simulink model "backups"  (R2024a)
settings: Solver=VariableStepAuto  StartTime=0.0  StopTime=10.0  RelTol=1e-3
values from neighbouring files (symbols this model uses):
  AttKd_x = inp(4,2).Var2    [SFF_Simulator_Entradas.m]
  AttKd_y = inp(5,2).Var2    [SFF_Simulator_Entradas.m]
  AttKd_z = inp(6,2).Var2    [SFF_Simulator_Entradas.m]
  AttKp_x = inp(1,2).Var2    [SFF_Simulator_Entradas.m]
  AttKp_y = inp(2,2).Var2    [SFF_Simulator_Entradas.m]
  AttKp_z = inp(3,2).Var2    [SFF_Simulator_Entradas.m]
  B = inp(8,2).Var2    [SFF_Simulator_Entradas.m]
  beta = inp(2,2).Var2    [SFF_Simulator_Entradas.m]
  Cd1 = inp(4,2).Var2    [SFF_Simulator_Entradas.m]
  cdgps = inp(1,2).Var2    [SFF_Simulator_Entradas.m]
  estrelas = inp(4,2).Var2    [SFF_Simulator_Entradas.m]
  estrelas_bias = inp(6,2).Var2    [SFF_Simulator_Entradas.m]
  estrelas_ruido = inp(5,2).Var2    [SFF_Simulator_Entradas.m]
  Fn = inp(2,2).Var2    [SFF_Simulator_Entradas.m]
  gps_bias = inp(3,2).Var2    [SFF_Simulator_Entradas.m]
  gps_ruido = inp(2,2).Var2    [SFF_Simulator_Entradas.m]
  Iw = inp(7,2).Var2    [SFF_Simulator_Entradas.m]
  Ixx = inp(7,2).Var2    [SFF_Simulator_Entradas.m]
  Iyy = inp(8,2).Var2    [SFF_Simulator_Entradas.m]
  Izz = inp(9,2).Var2    [SFF_Simulator_Entradas.m]
  Km = inp(3,2).Var2    [SFF_Simulator_Entradas.m]
  Kv = inp(9,2).Var2    [SFF_Simulator_Entradas.m]
  L1 = inp(5,2).Var2    [SFF_Simulator_Entradas.m]
  limCorrente = inp(4,2).Var2    [SFF_Simulator_Entradas.m]
  limVolt = inp(5,2).Var2    [SFF_Simulator_Entradas.m]
  m1 = inp(6,2).Var2    [SFF_Simulator_Entradas.m]
  magne = inp(10,2).Var2    [SFF_Simulator_Entradas.m]
  magne_bias = inp(12,2).Var2    [SFF_Simulator_Entradas.m]
  magne_ruido = inp(11,2).Var2    [SFF_Simulator_Entradas.m]
  man = inp(1,2).Var2    [SFF_Simulator_Entradas.m]
  OrbKd_x = inp(3,2).Var2    [SFF_Simulator_Entradas.m]
  OrbKd_y = inp(6,2).Var2    [SFF_Simulator_Entradas.m]
  OrbKd_z = inp(9,2).Var2    [SFF_Simulator_Entradas.m]
  OrbKi_x = inp(2,2).Var2    [SFF_Simulator_Entradas.m]
  OrbKi_y = inp(5,2).Var2    [SFF_Simulator_Entradas.m]
  OrbKi_z = inp(8,2).Var2    [SFF_Simulator_Entradas.m]
  OrbKp_x = inp(1,2).Var2    [SFF_Simulator_Entradas.m]
  OrbKp_y = inp(4,2).Var2    [SFF_Simulator_Entradas.m]
  OrbKp_z = inp(7,2).Var2    [SFF_Simulator_Entradas.m]
  propForcaAtivo = inp(1,2).Var2    [SFF_Simulator_Entradas.m]
  Rm = inp(6,2).Var2    [SFF_Simulator_Entradas.m]
  rodaAtivo = inp(1,2).Var2    [SFF_Simulator_Entradas.m]
  RodKi = inp(1,2).Var2    [SFF_Simulator_Entradas.m]
  sat_torquerod = inp(14,2).Var2    [SFF_Simulator_Entradas.m]
  torqrodAtivo = inp(1,2).Var2    [SFF_Simulator_Entradas.m]
undefined symbols (not defined in the file or in its folder): IAU, J2, mi, omega_E, propMomentoAtivo, Re, sat_rodareacao, WMM2020
libraries: dspsrcs4 x19, aerolibtransform2 x2, aerolibgravity2 x2, simulink x1
(part 3 of 4)

== system backups/Atuadores de Atitude/Atuador atitude ativado ==
  note: Entradas
  note: Atuador atitude ativado
  note: Saídas
  MtsProp : Inport
  Mts : Inport  Port=2
  dinCinOrb : Inport  Port=3
  A_q : Inport  Port=4
  Action Port : ActionPort  ActionPortLabel=if(u1 > 0)
  Bus Selector : BusSelector  OutputSignals=T_In_LVLH,r1_vec_I
  Cast To Single : DataTypeConversion  OutDataTypeStr=single  SaturateOnIntegerOverflow=off  RndMeth=Floor
  Cast To Single1 : DataTypeConversion  OutDataTypeStr=single  SaturateOnIntegerOverflow=off  RndMeth=Floor
  Cast To Single2 : DataTypeConversion  OutDataTypeStr=single  SaturateOnIntegerOverflow=off  RndMeth=Floor
  Constant4 : Constant  Value=rodaAtivo  SampleTime=-1
  Constant5 : Constant  Value=propForcaAtivo  SampleTime=-1
  Constant9 : Constant  Value=torqrodAtivo  SampleTime=-1
  If : If  NumInputs=3  IfExpression=u1 > 0 & u2 == 0 & u3 == 0  ElseIfExpressions=u2 > 0, u3 > 0  ShowElse=off
  Magnetorquer ativado : Subsystem  TreatAsAtomicUnit=on
  Merge : Merge  Inputs=3
  Propulsor ativado : Subsystem  TreatAsAtomicUnit=on
  Rodas de reação ativadas : Subsystem  TreatAsAtomicUnit=on
  MtsReal : Outport
  wires:
  Bus Selector/2 -> [r1_vec_I]  "<r1_vec_I>"
  Bus Selector/1 -> [T_In_LVLH]  "<T_In_LVLH>"
  dinCinOrb/1 -> Bus Selector/1
  If/1 -> Propulsor ativado/Action
  Propulsor ativado/1(Out1) -> Merge/1
  Rodas de reação ativadas/1(TcReal_rodareacao) -> Merge/2
  Magnetorquer ativado/1(TcReal_torqrod_roda) -> Merge/3
  If/3 -> Magnetorquer ativado/Action
  MtsProp/1 -> [MtsProp]
  Mts/1 -> [Mts]
  A_q/1 -> [A_q]
  Merge/1 -> [MtsReal]
  [MtsReal] -> MtsReal/1
  Constant9/1 -> Cast To Single2/1
  Cast To Single1/1 -> If/2
  Cast To Single2/1 -> If/3
  Constant4/1 -> Cast To Single1/1
  Cast To Single/1 -> If/1
  Constant5/1 -> Cast To Single/1
  [MtsProp] -> Propulsor ativado/1(In1)
  [Mts] -> Rodas de reação ativadas/1(Tc)
  If/2 -> Rodas de reação ativadas/Action
  [MtsProp] -> Rodas de reação ativadas/2(MtsProp)
  [A_q] -> Magnetorquer ativado/3(A_q)
  [T_In_LVLH] -> Magnetorquer ativado/2(T_In_LVLH)
  [r1_vec_I] -> Magnetorquer ativado/4(r1_vec_I)
  [Mts] -> Magnetorquer ativado/1(Tc)
  [MtsProp] -> Magnetorquer ativado/5(MtsProp)

== system backups/Atuadores de Atitude/Atuador atitude desativado ==
  In1 : Inport
  Action Port : ActionPort  ActionPortLabel=else
  Out1 : Outport
  wires:
  In1/1 -> Out1/1

== system backups/Atuadores de Atitude1/Atuador atitude ativado ==
  note: Entradas
  note: Atuador atitude ativado
  note: Saídas
  MtsProp : Inport
  Mts : Inport  Port=2
  dinCinOrb : Inport  Port=3
  A_q : Inport  Port=4
  Action Port : ActionPort
  Bus Selector : BusSelector  OutputSignals=T_In_LVLH,r1_vec_I
  Cast To Single : DataTypeConversion  OutDataTypeStr=single  SaturateOnIntegerOverflow=off  RndMeth=Floor
  Cast To Single1 : DataTypeConversion  OutDataTypeStr=single  SaturateOnIntegerOverflow=off  RndMeth=Floor
  Cast To Single2 : DataTypeConversion  OutDataTypeStr=single  SaturateOnIntegerOverflow=off  RndMeth=Floor
  Constant4 : Constant  Value=rodaAtivo  SampleTime=-1
  Constant5 : Constant  Value=propForcaAtivo  SampleTime=-1
  Constant9 : Constant  Value=torqrodAtivo  SampleTime=-1
  If : If  NumInputs=3  IfExpression=u1 > 0 & u2 == 0 & u3 == 0  ElseIfExpressions=u2 > 0, u3 > 0  ShowElse=off
  Magnetorquer ativado : Subsystem  TreatAsAtomicUnit=on
  Merge : Merge  Inputs=3
  Propulsor ativado : Subsystem  TreatAsAtomicUnit=on
  Rodas de reação ativadas : Subsystem  TreatAsAtomicUnit=on
  MtsReal : Outport
  wires:
  Bus Selector/2 -> [r1_vec_I]  "<r1_vec_I>"
  Bus Selector/1 -> [T_In_LVLH]  "<T_In_LVLH>"
  dinCinOrb/1 -> Bus Selector/1
  Constant5/1 -> Cast To Single/1
  Cast To Single/1 -> If/1
  Constant4/1 -> Cast To Single1/1
  Constant9/1 -> Cast To Single2/1
  Cast To Single1/1 -> If/2
  Cast To Single2/1 -> If/3
  If/1 -> Propulsor ativado/Action
  If/2 -> Rodas de reação ativadas/Action
  Propulsor ativado/1(Out1) -> Merge/1
  Rodas de reação ativadas/1(TcReal_rodareacao) -> Merge/2
  Magnetorquer ativado/1(TcReal_torqrod_roda) -> Merge/3
  If/3 -> Magnetorquer ativado/Action
  MtsProp/1 -> [MtsProp]
  [MtsProp] -> Propulsor ativado/1(In1)
  Mts/1 -> [Mts]
  [Mts] -> Magnetorquer ativado/1(Tc)
  [T_In_LVLH] -> Magnetorquer ativado/2(T_In_LVLH)
  [r1_vec_I] -> Magnetorquer ativado/4(r1_vec_I)
  [A_q] -> Magnetorquer ativado/3(A_q)
  A_q/1 -> [A_q]
  Merge/1 -> [MtsReal]
  [MtsReal] -> MtsReal/1
  [Mts] -> Rodas de reação ativadas/1(Tc)
  [MtsProp] -> Rodas de reação ativadas/2(MtsProp)
  [MtsProp] -> Magnetorquer ativado/5(MtsProp)

== system backups/Atuadores de Atitude1/Atuador atitude desativado ==
  In1 : Inport
  Action Port : ActionPort
  Out1 : Outport
  wires:
  In1/1 -> Out1/1

== system backups/Sensores Atitude/Sensor ativado ==
  atitudeIn : Inport
  Action Port : ActionPort
  Demux : Demux  Outputs=3
  Mux : Mux  Inputs=3
  estrelasSensor_phi : Subsystem
  estrelasSensor_psi : Subsystem
  estrelasSensor_theta : Subsystem
  atitudeOut : Outport
  wires:
  Demux/3 -> estrelasSensor_psi/1(In1)
  Demux/2 -> estrelasSensor_theta/1(In1)
  Demux/1 -> estrelasSensor_phi/1(phiIn)
  atitudeIn/1 -> Demux/1
  estrelasSensor_phi/1(phiOut) -> Mux/1
  estrelasSensor_theta/1(Out1) -> Mux/2
  estrelasSensor_psi/1(Out1) -> Mux/3
  Mux/1 -> atitudeOut/1

== system backups/Sensores Atitude/Sensor desativado ==
  atitudeIn : Inport
  Action Port : ActionPort
  atitudeOut : Outport
  wires:
  atitudeIn/1 -> atitudeOut/1

== system backups/Sensores Atitude1/Sensor ativado ==
  atitude : Inport
  Action Port : ActionPort
  Demux : Demux  Outputs=3
  Mux : Mux  Inputs=3
  estrelasSensor_phi : Subsystem
  estrelasSensor_psi : Subsystem
  estrelasSensor_theta : Subsystem
  atitudeSen : Outport
  wires:
  Demux/3 -> estrelasSensor_psi/1(In1)
  Demux/2 -> estrelasSensor_theta/1(In1)
  Demux/1 -> estrelasSensor_phi/1(In1)
  atitude/1 -> Demux/1
  estrelasSensor_phi/1(Out1) -> Mux/1  "x"
  estrelasSensor_theta/1(Out1) -> Mux/2  "y"
  estrelasSensor_psi/1(Out1) -> Mux/3  "z"
  Mux/1 -> atitudeSen/1

== system backups/Sensores Atitude1/Sensor desativado ==
  atitude : Inport
  Action Port : ActionPort
  atitudeSen : Outport
  wires:
  atitude/1 -> atitudeSen/1

== system backups/Sensores Orbital/Sensor ativado ==
  dinCinOrbIn : Inport
  Action Port : ActionPort
  Bus Creator : BusCreator  Inputs=18
  Bus Selector : BusSelector  OutputSignals=x,y,z
  Bus Selector1 : BusSelector  OutputSignals=x_dot,y_dot,z_dot,r0,omega_x,omega_y,omega_z,omega_x_dot,omega_y_dot,omega_z_dot,T_In_LVLH,r1_vec_I,i1,ohm1,theta1
  GPSsensor : Subsystem
  GPSsensor1 : Subsystem
  GPSsensor2 : Subsystem
  dinCinOrbOut : Outport
  wires:
  Bus Selector/3 -> GPSsensor2/1(In1)  "<z>"
  Bus Selector/2 -> GPSsensor1/1(In1)  "<y>"
  Bus Selector/1 -> GPSsensor/1(In1)  "<x>"
  dinCinOrbIn/1 -> Bus Selector/1, Bus Selector1/1
  Bus Creator/1 -> dinCinOrbOut/1
  Bus Selector1/4 -> Bus Creator/7  "<r0>"
  Bus Selector1/5 -> Bus Creator/8  "<omega_x>"
  Bus Selector1/6 -> Bus Creator/9  "<omega_y>"
  Bus Selector1/7 -> Bus Creator/10  "<omega_z>"
  Bus Selector1/8 -> Bus Creator/11  "<omega_x_dot>"
  Bus Selector1/9 -> Bus Creator/12  "<omega_y_dot>"
  Bus Selector1/10 -> Bus Creator/13  "<omega_z_dot>"
  Bus Selector1/11 -> Bus Creator/14  "<T_In_LVLH>"
  Bus Selector1/12 -> Bus Creator/15  "<r1_vec_I>"
  Bus Selector1/13 -> Bus Creator/16  "<i1>"
  Bus Selector1/14 -> Bus Creator/17  "<ohm1>"
  Bus Selector1/15 -> Bus Creator/18  "<theta1>"
  GPSsensor2/1(Out1) -> Bus Creator/5  "z"
  GPSsensor1/1(Out1) -> Bus Creator/3  "y"
  GPSsensor/1(Out1) -> Bus Creator/1  "x"
  Bus Selector1/1 -> Bus Creator/2  "<x_dot>"
  Bus Selector1/2 -> Bus Creator/4  "<y_dot>"
  Bus Selector1/3 -> Bus Creator/6  "<z_dot>"

== system backups/Sensores Orbital/Sensor desativado ==
  dinCinOrbIn : Inport
  Action Port : ActionPort
  dinCinOrbOut : Outport
  wires:
  dinCinOrbIn/1 -> dinCinOrbOut/1

== system backups/Sensores Orbital1/Sensor ativado ==
  dinCinOrb : Inport
  Action Port : ActionPort
  Bus Creator : BusCreator  Inputs=18
  Bus Selector : BusSelector  OutputSignals=x,y,z
  Bus Selector1 : BusSelector  OutputSignals=x_dot,y_dot,z_dot,r0,omega_x,omega_y,omega_z,omega_x_dot,omega_y_dot,omega_z_dot,T_In_LVLH,r1_vec_I,i1,ohm1,theta1
  GPSsensor : Subsystem
  GPSsensor1 : Subsystem
  GPSsensor2 : Subsystem
  Out1 : Outport
  wires:
  Bus Selector/3 -> GPSsensor2/1(In1)  "<z>"
  Bus Selector/2 -> GPSsensor1/1(In1)  "<y>"
  Bus Selector/1 -> GPSsensor/1(In1)  "<x>"
  dinCinOrb/1 -> Bus Selector/1, Bus Selector1/1
  Bus Creator/1 -> Out1/1
  Bus Selector1/4 -> Bus Creator/7  "<r0>"
  Bus Selector1/5 -> Bus Creator/8  "<omega_x>"
  Bus Selector1/6 -> Bus Creator/9  "<omega_y>"
  Bus Selector1/7 -> Bus Creator/10  "<omega_z>"
  Bus Selector1/8 -> Bus Creator/11  "<omega_x_dot>"
  Bus Selector1/9 -> Bus Creator/12  "<omega_y_dot>"
  Bus Selector1/10 -> Bus Creator/13  "<omega_z_dot>"
  Bus Selector1/11 -> Bus Creator/14  "<T_In_LVLH>"
  Bus Selector1/12 -> Bus Creator/15  "<r1_vec_I>"
  Bus Selector1/13 -> Bus Creator/16  "<i1>"
  Bus Selector1/14 -> Bus Creator/17  "<ohm1>"
  Bus Selector1/15 -> Bus Creator/18  "<theta1>"
  GPSsensor2/1(Out1) -> Bus Creator/5  "z"
  GPSsensor1/1(Out1) -> Bus Creator/3  "y"
  GPSsensor/1(Out1) -> Bus Creator/1  "x"
  Bus Selector1/1 -> Bus Creator/2  "<x_dot>"
  Bus Selector1/2 -> Bus Creator/4  "<y_dot>"
  Bus Selector1/3 -> Bus Creator/6  "<z_dot>"

== system backups/Sensores Orbital1/Sensor desativado ==
  dinCinOrb : Inport
  Action Port : ActionPort
  Out1 : Outport
  wires:
  dinCinOrb/1 -> Out1/1

== system backups/atuadoresAtitude/conjunto2TorqRods1RodaReacao ==
  Tc : Inport
  T_In_LVLH : Inport  Port=2
  A_q : Inport  Port=3
  r1_vec_I : Inport  Port=4
  Constant9 : Constant  Value=torqrodAtivo  SampleTime=-1
  Demux1 : Demux  Outputs=3
  ECI Position to LLA : aerolibtransform2/ECI Position to LLA  red=IAU-2000/2006  year=2013  month=January  day=1  hour=0  min=0  sec=0  deltaT=None  errorflag=Error  extraparamflag=off  eunits=Metric (MKS)  earthmodel=WGS84  flat=1/298.257223563  eqradius=6378137
      settings: AttributesFormatString=%<red>
  Gain : Gain  Gain=pi/180
  Gain1 : Gain  Gain=pi/180
  HardwareDeControle (Rodas de Reação + 2 Torqrods) : Subsystem
  If : If
  If Action Subsystem : Subsystem  TreatAsAtomicUnit=on
  If Action Subsystem1 : Subsystem  TreatAsAtomicUnit=on
  Merge : Merge
  Product : Product  Multiplication=Matrix(*)
  Product1 : Product  Multiplication=Matrix(*)
  TcReal_torqrod_roda : Outport
  wires:
  HardwareDeControle (Rodas de Reação + 2 Torqrods)/1(Tc fornecido) -> TcReal_torqrod_roda/1
  Tc/1 -> HardwareDeControle (Rodas de Reação + 2 Torqrods)/1(Tc)
  T_In_LVLH/1 -> Product/1
  Product/1 -> Product1/2
  Product1/1 -> HardwareDeControle (Rodas de Reação + 2 Torqrods)/2(B_seg)  "B_seg"
  A_q/1 -> Product1/1
  Constant9/1 -> [torqrodAtivo]
  [torqrodAtivo] -> If/1
  If/1 -> If Action Subsystem/Action
  [lonSeg] -> If Action Subsystem/3(lonSeg)
  [altSeg] -> If Action Subsystem/1(altSeg)
  [latSeg] -> If Action Subsystem/2(latSeg)
  If/2 -> If Action Subsystem1/Action
  If Action Subsystem/1(Output) -> Merge/1
  If Action Subsystem1/1(Out1) -> Merge/2
  Merge/1 -> Product/2
  Demux1/3 -> [altSeg]
  Gain1/1 -> [lonSeg]
  Demux1/2 -> Gain1/1
  Demux1/1 -> Gain/1
  ECI Position to LLA/1 -> Demux1/1
  Gain/1 -> [latSeg]
  r1_vec_I/1 -> ECI Position to LLA/1

== system backups/atuadoresAtitude/rodaReacao ==
  note: Acelerações e velocidades angulares de cada roda estão contidas dentro do bloco rodaReacaoCaracteristicas
  Tc : Inport
  Acelerações angulares de cada roda : Scope
  Aw*u : Gain  Gain=[1 0 -1 0; 0 1 0 -1; 1 1 1 1; 1 -1 1 -1]  Multiplication=Matrix(K*u)
  Constant : Constant  Value=0  SampleTime=-1
  Demux : Demux  Outputs=3
  Demux1 : Demux
  Demux2 : Demux
  Gain1 : Gain  Gain=1/cos(beta)
  Gain10 : Gain  Gain=1/sin(beta)
  Gain12 : Gain  Gain=1/Iw
  Gain2 : Gain  Gain=cos(beta)
  Gain3 : Gain  Gain=sin(beta)
  Gain4 : Gain  Gain=cos(beta)
  Gain9 : Gain  Gain=1/cos(beta)
  Integrator : Integrator  InitialCondition=[0 0 0 0]
  Mux : Mux
  Mux1 : Mux
  Mux2 : Mux  Inputs=3
  Scope1 : Scope
  T1 T2 T3 T4 : Scope
  Terminator : Terminator
  Torques fornecidos por cada roda de reação : Scope
  Torques requisitados para cada roda de reação : Scope
  Velocidades angulares de cada roda : Scope
  inv(Aw)*u : Gain  Gain=0.5*[1 0 0.5 0.5;0 1 0.5 -0.5; -1 0 0.5 0.5; 0 -1 0.5 -0.5]  Multiplication=Matrix(K*u)
  rodaReacaoCaracteristicas : Subsystem
  rodaReacaoCaracteristicas1 : Subsystem
  rodaReacaoCaracteristicas2 : Subsystem
  rodaReacaoCaracteristicas3 : Subsystem
  TcReal_rodareacao : Outport
  wires:
  Demux/1 -> Gain1/1
  Demux/3 -> Gain10/1
  Tc/1 -> Demux/1
  Gain9/1 -> Mux/2
  Gain12/1 -> Integrator/1, Acelerações angulares de cada roda/1
  Constant/1 -> Mux/4
  Demux/2 -> Gain9/1
  Gain1/1 -> Mux/1
  Gain10/1 -> Mux/3
  Integrator/1 -> Velocidades angulares de cada roda/1
  Mux/1 -> inv(Aw)*u/1
  inv(Aw)*u/1 -> Torques requisitados para cada roda de reação/1, Demux1/1  "T1 T2 T3 T4"
  Mux1/1 -> Torques fornecidos por cada roda de reação/1, Aw*u/1, Gain12/1
  Demux1/1 -> rodaReacaoCaracteristicas/1(Tc_entrada)
  Demux1/2 -> rodaReacaoCaracteristicas1/1(Tc_entrada)
  Demux1/3 -> rodaReacaoCaracteristicas2/1(Tc_entrada)
  Demux1/4 -> rodaReacaoCaracteristicas3/1(Tc_entrada)
  rodaReacaoCaracteristicas3/1(Tw) -> Mux1/4
  rodaReacaoCaracteristicas2/1(Tw) -> Mux1/3
  rodaReacaoCaracteristicas1/1(Tw) -> Mux1/2
  rodaReacaoCaracteristicas/1(Tw) -> Mux1/1
  Aw*u/1 -> Demux2/1, T1 T2 T3 T4/1  "T1 T2 T3 T4"
  Demux2/3 -> Gain3/1
  Demux2/2 -> Gain4/1
  Demux2/1 -> Gain2/1
  Demux2/4 -> Terminator/1
  Mux2/1 -> Scope1/1, TcReal_rodareacao/1
  Gain2/1 -> Mux2/1
  Gain4/1 -> Mux2/2
  Gain3/1 -> Mux2/3

== system backups/Atuadores Orbital1/Propulsor ativado/If Action Subsystem ==
  In1 : Inport
  Action Port : ActionPort
  Out1 : Outport
  wires:
  In1/1 -> Out1/1

== system backups/Atuadores Orbital1/Propulsor ativado/If Action Subsystem1 ==
  In1 : Inport
  Action Port : ActionPort
  Out1 : Outport
  wires:
  In1/1 -> Out1/1

== system backups/Atuadores de Atitude/Atuador atitude ativado/Magnetorquer ativado ==
  note: Magnetotorqueador
  note: Saídas
  note: Entradas
  Tc : Inport
  T_In_LVLH : Inport  Port=2
  A_q : Inport  Port=3
  r1_vec_I : Inport  Port=4
  MtsProp : Inport  Port=5
  Action Port : ActionPort  ActionPortLabel=elseif( u3 > 0)
  Add : Sum
  Conjunto Rodas de Reação + Magnetotorques : Subsystem
  Demux1 : Demux  Outputs=3
  ECI Position to LLA : aerolibtransform2/ECI Position to LLA  red=IAU-2000/2006  year=2013  month=January  day=1  hour=0  min=0  sec=0  deltaT=None  errorflag=Error  extraparamflag=off  eunits=Metric (MKS)  earthmodel=WGS84  flat=1/298.257223563  eqradius=6378137
      settings: AttributesFormatString=%<red>
  Gain2 : Gain  Gain=1e-9
  Magnetômetro : Subsystem
  Product : Product  Multiplication=Matrix(*)
  Product1 : Product  Multiplication=Matrix(*)
  Unit Delay : UnitDelay  SampleTime=-1  HasFrameUpgradeWarning=on
  World Magnetic Model : aerolibgravity2/World Magnetic Model  model=WMM2020 (2020-2025)  customFile='WMM2020.COF'  units=Metric (MKS)  time_in=off  month=January  day=1  year=2024  action=Error  h_out=off  dec_out=off  inc_out=off  ti_out=off
  TcReal_torqrod_roda : Outport
  wires:
  Demux1/2 -> [lonSeg]
  Product/1 -> Product1/2
  Demux1/1 -> [latSeg]
  Demux1/3 -> [altSeg]
  Product1/1 -> Conjunto Rodas de Reação + Magnetotorques/2(B_seg)  "B_seg"
  Unit Delay/1 -> Product1/1
  [Tc] -> Conjunto Rodas de Reação + Magnetotorques/1(Tc)
  [A_q] -> Unit Delay/1
  [T_In_LVLH] -> Product/1
  Conjunto Rodas de Reação + Magnetotorques/1(Tc_real) -> [TcReal_torqrod_roda]
  Magnetômetro/1(B_sen) -> [B_sen]
  [B] -> Magnetômetro/1(B)
  Gain2/1 -> [B]
  [B_sen] -> Product/2
  [r1_vec_I] -> ECI Position to LLA/1
  ECI Position to LLA/1 -> Demux1/1
  [TcReal_torqrod_roda] -> Add/1
  [MtsProp] -> Add/2
  Add/1 -> TcReal_torqrod_roda/1
  T_In_LVLH/1 -> [T_In_LVLH]
  r1_vec_I/1 -> [r1_vec_I]
  MtsProp/1 -> [MtsProp]
  A_q/1 -> [A_q]
  Tc/1 -> [Tc]
  World Magnetic Model/1 -> Gain2/1
  [lonSeg] -> World Magnetic Model/3
  [latSeg] -> World Magnetic Model/2
  [altSeg] -> World Magnetic Model/1

== system backups/Atuadores de Atitude/Atuador atitude ativado/Propulsor ativado ==
  In1 : Inport
  Action Port : ActionPort  ActionPortLabel=if(u1 > 0 & u2 == 0 & u3 == 0)
  Out1 : Outport
  wires:
  In1/1 -> Out1/1

== system backups/Atuadores de Atitude/Atuador atitude ativado/Rodas de reação ativadas ==
  note: Rodas de Reação
  note: Entradas
  note: Saídas
  Tc : Inport
  MtsProp : Inport  Port=2
  Action Port : ActionPort  ActionPortLabel=elseif(u2 > 0)
  Add : Sum
  Aw*u : Gain  Gain=[1 0 -1 0; 0 1 0 -1; 1 1 1 1; 1 -1 1 -1]  Multiplication=Matrix(K*u)
  Constant : Constant  Value=0  SampleTime=-1
  Demux : Demux  Outputs=3
  Demux1 : Demux
  Demux2 : Demux
  Gain1 : Gain  Gain=1/cos(beta)
  Gain10 : Gain  Gain=1/sin(beta)
  Gain2 : Gain  Gain=cos(beta)
  Gain3 : Gain  Gain=sin(beta)
  Gain4 : Gain  Gain=cos(beta)
  Gain5 : Gain  Gain=1/cos(beta)
  Mux : Mux
  Mux1 : Mux
  Mux2 : Mux  Inputs=3
  Terminator : Terminator
  i : Gain  Gain=0.5*[1 0 0.5 0.5;0 1 0.5 -0.5; -1 0 0.5 0.5; 0 -1 0.5 -0.5]  Multiplication=Matrix(K*u)
  rodaReacaoCaracteristicas{,1..2,4} (4 alike) : ModelReference  ModelNameDialog=rodaReacaoCaracteristicas  ModelReferenceVersion=3.129
  TcReal_rodareacao : Outport
  wires:
  Mux2/1 -> [TcReal_rodareacao]
  rodaReacaoCaracteristicas2/1 -> Mux1/4
  Constant/1 -> Mux/4
  Mux/1 -> i/1
  Gain2/1 -> Mux2/1
  Demux2/1 -> Gain2/1
  Gain1/1 -> Mux/1
  Gain4/1 -> Mux2/2
  Demux2/4 -> Terminator/1
  Gain3/1 -> Mux2/3
  Gain10/1 -> Mux/3
  Mux1/1 -> Aw*u/1
  i/1 -> Demux1/1
  Demux/2 -> Gain5/1
  Demux2/3 -> Gain3/1
  rodaReacaoCaracteristicas1/1 -> Mux1/3
  Aw*u/1 -> Demux2/1
  Gain5/1 -> Mux/2
  rodaReacaoCaracteristicas/1 -> Mux1/1
  Demux/3 -> Gain10/1
  Demux/1 -> Gain1/1
  rodaReacaoCaracteristicas4/1 -> Mux1/2
  Demux2/2 -> Gain4/1
  Tc/1 -> [Tc]
  [Tc] -> Demux/1
  Demux1/4 -> rodaReacaoCaracteristicas2/1
  Demux1/3 -> rodaReacaoCaracteristicas1/1
  Demux1/2 -> rodaReacaoCaracteristicas4/1
  Demux1/1 -> rodaReacaoCaracteristicas/1
  [TcReal_rodareacao] -> Add/1
  [MtsProp] -> Add/2
  Add/1 -> TcReal_rodareacao/1
  MtsProp/1 -> [MtsProp]

== system backups/Atuadores de Atitude1/Atuador atitude ativado/Magnetorquer ativado ==
  note: Magnetorquer
  note: Saídas
  note: Entradas
  Tc : Inport
  T_In_LVLH : Inport  Port=2
  A_q : Inport  Port=3
  r1_vec_I : Inport  Port=4
  MtsProp : Inport  Port=5
  Action Port : ActionPort
  Add : Sum
  Constant : Constant  Value=1.5*10^-5
  Constant1 : Constant  Value=-10*10^-7
  Constant2 : Constant  Value=3.5*10^-5
  HardwareDeControle (Rodas de Reação + 2 Torqrods) : Subsystem
  Magnetômetro : Subsystem
  Mux : Mux  Inputs=3
  Product : Product  Multiplication=Matrix(*)
  Product1 : Product  Multiplication=Matrix(*)
  Unit Delay : UnitDelay  SampleTime=-1  HasFrameUpgradeWarning=on
  TcReal_torqrod_roda : Outport
  wires:
  Product/1 -> Product1/2
  Product1/1 -> HardwareDeControle (Rodas de Reação + 2 Torqrods)/2(B_seg)  "B_seg"
  Unit Delay/1 -> Product1/1
  Tc/1 -> [Tc]
  T_In_LVLH/1 -> [T_In_LVLH]
  A_q/1 -> [A_q]
  r1_vec_I/1 -> [r1_vec_I]
  [Tc] -> HardwareDeControle (Rodas de Reação + 2 Torqrods)/1(Tc)
  [A_q] -> Unit Delay/1
  [T_In_LVLH] -> Product/1
  HardwareDeControle (Rodas de Reação + 2 Torqrods)/1(Tc fornecido) -> [TcReal_torqrod_roda]
  Magnetômetro/1(B_sen) -> [B_sen]
  [B] -> Magnetômetro/1(B)
  Mux/1 -> [B]
  [B_sen] -> Product/2
  Constant/1 -> Mux/1
  Constant1/1 -> Mux/2
  Constant2/1 -> Mux/3
  [MtsProp] -> Add/2
  [TcReal_torqrod_roda] -> Add/1
  Add/1 -> TcReal_torqrod_roda/1
  MtsProp/1 -> [MtsProp]

== system backups/Atuadores de Atitude1/Atuador atitude ativado/Propulsor ativado ==
  In1 : Inport
  Action Port : ActionPort
  Out1 : Outport
  wires:
  In1/1 -> Out1/1

== system backups/Atuadores de Atitude1/Atuador atitude ativado/Rodas de reação ativadas ==
  note: Rodas de Reação
  note: Entradas
  note: Saídas
  Tc : Inport
  MtsProp : Inport  Port=2
  Action Port : ActionPort
  Add : Sum
  Aw*u : Gain  Gain=[1 0 -1 0; 0 1 0 -1; 1 1 1 1; 1 -1 1 -1]  Multiplication=Matrix(K*u)
  Constant : Constant  Value=0  SampleTime=-1
  Demux : Demux  Outputs=3
  Demux1 : Demux
  Demux2 : Demux
  Gain1 : Gain  Gain=1/cos(beta)
  Gain10 : Gain  Gain=1/sin(beta)
  Gain2 : Gain  Gain=cos(beta)
  Gain3 : Gain  Gain=sin(beta)
  Gain4 : Gain  Gain=cos(beta)
  Gain9 : Gain  Gain=1/cos(beta)
  Mux : Mux
  Mux1 : Mux
  Mux2 : Mux  Inputs=3
  Terminator : Terminator
  i : Gain  Gain=0.5*[1 0 0.5 0.5;0 1 0.5 -0.5; -1 0 0.5 0.5; 0 -1 0.5 -0.5]  Multiplication=Matrix(K*u)
  rodaReacaoCaracteristicas{,1..2,4} (4 alike) : ModelReference  ModelNameDialog=rodaReacaoCaracteristicas  ModelReferenceVersion=3.129
  TcReal_rodareacao : Outport
  wires:
  Mux2/1 -> [TcReal_rodareacao]
  rodaReacaoCaracteristicas2/1 -> Mux1/4
  Constant/1 -> Mux/4
  Mux/1 -> i/1
  Gain2/1 -> Mux2/1
  Demux2/1 -> Gain2/1
  Gain1/1 -> Mux/1
  Gain4/1 -> Mux2/2
  Demux2/4 -> Terminator/1
  Gain3/1 -> Mux2/3
  Gain10/1 -> Mux/3
  Mux1/1 -> Aw*u/1
  i/1 -> Demux1/1
  Demux/2 -> Gain9/1
  Demux2/3 -> Gain3/1
  rodaReacaoCaracteristicas1/1 -> Mux1/3
  Aw*u/1 -> Demux2/1
  Gain9/1 -> Mux/2
  rodaReacaoCaracteristicas/1 -> Mux1/1
  Demux/3 -> Gain10/1
  Demux/1 -> Gain1/1
  rodaReacaoCaracteristicas4/1 -> Mux1/2
  Demux2/2 -> Gain4/1
  Tc/1 -> [Tc]
  [Tc] -> Demux/1
  Demux1/4 -> rodaReacaoCaracteristicas2/1
  Demux1/3 -> rodaReacaoCaracteristicas1/1
  Demux1/2 -> rodaReacaoCaracteristicas4/1
  Demux1/1 -> rodaReacaoCaracteristicas/1
  [TcReal_rodareacao] -> Add/1
  [MtsProp] -> Add/2
  Add/1 -> TcReal_rodareacao/1
  MtsProp/1 -> [MtsProp]

== system backups/Sensores Atitude/Sensor ativado/estrelasSensor_phi ==
  phiIn : Inport
  Add1 : Sum
  Add2 : Sum
  Ruído : dspsrcs4/Random Source  SrcType=Uniform  MinVal=-estrelas_ruido  MaxVal=estrelas_ruido  MeanVal=0  VarVal=1  RepMode=Not repeatable  rawSeed=1  IsInherit=off  SampTime=step_modelo  SampFrame=1  OutComplex=Real  DataType=double  SimulateUsing=Code generation
  Viés : Constant  Value=estrelas_bias
  phiOut : Outport
  wires:
  Ruído/1 -> Add2/1
  phiIn/1 -> Add1/2
  Viés/1 -> Add1/1
  Add1/1 -> Add2/2
  Add2/1 -> phiOut/1

== system backups/Sensores Atitude/Sensor ativado/estrelasSensor_psi ==
  In1 : Inport
  Add1 : Sum
  Add2 : Sum
  Constant : Constant  Value=estrelas_bias
  Random Source1 : dspsrcs4/Random Source  SrcType=Uniform  MinVal=-estrelas_ruido  MaxVal=estrelas_ruido  MeanVal=0  VarVal=1  RepMode=Not repeatable  rawSeed=1  IsInherit=off  SampTime=step_modelo  SampFrame=1  OutComplex=Real  DataType=double  SimulateUsing=Code generation
  Out1 : Outport
  wires:
  Random Source1/1 -> Add2/1
  Constant/1 -> Add1/1
  Add2/1 -> Out1/1
  In1/1 -> Add1/2
  Add1/1 -> Add2/2

== system backups/Sensores Atitude/Sensor ativado/estrelasSensor_theta ==
  In1 : Inport
  Add1 : Sum
  Add2 : Sum
  Constant : Constant  Value=estrelas_bias
  Random Source1 : dspsrcs4/Random Source  SrcType=Uniform  MinVal=-estrelas_ruido  MaxVal=estrelas_ruido  MeanVal=0  VarVal=1  RepMode=Not repeatable  rawSeed=1  IsInherit=off  SampTime=step_modelo  SampFrame=1  OutComplex=Real  DataType=double  SimulateUsing=Code generation
  Out1 : Outport
  wires:
  Random Source1/1 -> Add2/1
  Constant/1 -> Add1/1
  Add2/1 -> Out1/1
  In1/1 -> Add1/2
  Add1/1 -> Add2/2

== system backups/Sensores Atitude1/Sensor ativado/estrelasSensor_phi ==
  In1 : Inport
  Add1 : Sum
  Add2 : Sum
  Constant : Constant  Value=estrelas_bias*4.8481*10^-6
  Random Source1 : dspsrcs4/Random Source  SrcType=Uniform  MinVal=-estrelas_ruido*4.8481*10^-6  MaxVal=estrelas_ruido*4.8481*10^-6  MeanVal=0  VarVal=1  RepMode=Not repeatable  rawSeed=1  IsInherit=off  SampTime=step_modelo  SampFrame=1  OutComplex=Real  DataType=double  SimulateUsing=Code generation
  Out1 : Outport
  wires:
  Random Source1/1 -> Add2/1
  In1/1 -> Add1/2
  Constant/1 -> Add1/1
  Add1/1 -> Add2/2
  Add2/1 -> Out1/1

== system backups/Sensores Atitude1/Sensor ativado/estrelasSensor_psi ==
  In1 : Inport
  Add1 : Sum
  Add2 : Sum
  Constant : Constant  Value=estrelas_bias*4.8481*10^-6
  Random Source1 : dspsrcs4/Random Source  SrcType=Uniform  MinVal=-estrelas_ruido*4.8481*10^-6  MaxVal=estrelas_ruido*4.8481*10^-6  MeanVal=0  VarVal=1  RepMode=Not repeatable  rawSeed=1  IsInherit=off  SampTime=step_modelo  SampFrame=1  OutComplex=Real  DataType=double  SimulateUsing=Code generation
  Out1 : Outport
  wires:
  Random Source1/1 -> Add2/1
  Constant/1 -> Add1/1
  Add2/1 -> Out1/1
  In1/1 -> Add1/2
  Add1/1 -> Add2/2

== system backups/Sensores Atitude1/Sensor ativado/estrelasSensor_theta ==
  In1 : Inport
  Add1 : Sum
  Add2 : Sum
  Constant : Constant  Value=estrelas_bias*4.8481*10^-6
  Random Source1 : dspsrcs4/Random Source  SrcType=Uniform  MinVal=-estrelas_ruido*4.8481*10^-6  MaxVal=estrelas_ruido*4.8481*10^-6  MeanVal=0  VarVal=1  RepMode=Not repeatable  rawSeed=1  IsInherit=off  SampTime=step_modelo  SampFrame=1  OutComplex=Real  DataType=double  SimulateUsing=Code generation
  Out1 : Outport
  wires:
  Random Source1/1 -> Add2/1
  Constant/1 -> Add1/1
  Add2/1 -> Out1/1
  In1/1 -> Add1/2
  Add1/1 -> Add2/2

== system backups/Sensores Orbital/Sensor ativado/GPSsensor ==
  In1 : Inport
  Add1 : Sum
  Add2 : Sum
  Constant : Constant  Value=gps_bias
  Random Source1 : dspsrcs4/Random Source  SrcType=Uniform  MinVal=-gps_ruido  MaxVal=gps_ruido  MeanVal=0  VarVal=1  RepMode=Not repeatable  rawSeed=1  IsInherit=off  SampTime=step_modelo  SampFrame=1  OutComplex=Real  DataType=double  SimulateUsing=Code generation
  Out1 : Outport
  wires:
  Random Source1/1 -> Add2/1
  In1/1 -> Add1/2
  Constant/1 -> Add1/1
  Add1/1 -> Add2/2
  Add2/1 -> Out1/1

== system backups/Sensores Orbital/Sensor ativado/GPSsensor1 ==
  In1 : Inport
  Add1 : Sum
  Add2 : Sum
  Constant : Constant  Value=gps_bias
  Random Source1 : dspsrcs4/Random Source  SrcType=Uniform  MinVal=-gps_ruido  MaxVal=gps_ruido  MeanVal=0  VarVal=1  RepMode=Not repeatable  rawSeed=1  IsInherit=off  SampTime=step_modelo  SampFrame=1  OutComplex=Real  DataType=double  SimulateUsing=Code generation
  Out1 : Outport
  wires:
  Random Source1/1 -> Add2/1
  Constant/1 -> Add1/1
  Add1/1 -> Add2/2
  In1/1 -> Add1/2
  Add2/1 -> Out1/1

== system backups/Sensores Orbital/Sensor ativado/GPSsensor2 ==
  In1 : Inport
  Add1 : Sum
  Add2 : Sum
  Constant : Constant  Value=gps_bias
  Random Source1 : dspsrcs4/Random Source  SrcType=Uniform  MinVal=-gps_ruido  MaxVal=gps_ruido  MeanVal=0  VarVal=1  RepMode=Not repeatable  rawSeed=1  IsInherit=off  SampTime=step_modelo  SampFrame=1  OutComplex=Real  DataType=double  SimulateUsing=Code generation
  Out1 : Outport
  wires:
  Random Source1/1 -> Add2/1
  Constant/1 -> Add1/1
  Add1/1 -> Add2/2
  In1/1 -> Add1/2
  Add2/1 -> Out1/1

== system backups/Sensores Orbital1/Sensor ativado/GPSsensor ==
  In1 : Inport
  Add1 : Sum
  Add2 : Sum
  Constant : Constant  Value=gps_bias
  Random Source1 : dspsrcs4/Random Source  SrcType=Uniform  MinVal=-gps_ruido  MaxVal=gps_ruido  MeanVal=0  VarVal=1  RepMode=Not repeatable  rawSeed=1  IsInherit=off  SampTime=step_modelo  SampFrame=1  OutComplex=Real  DataType=double  SimulateUsing=Code generation
  Out1 : Outport
  wires:
  Random Source1/1 -> Add2/1
  In1/1 -> Add1/2
  Constant/1 -> Add1/1
  Add1/1 -> Add2/2
  Add2/1 -> Out1/1

== system backups/Sensores Orbital1/Sensor ativado/GPSsensor1 ==
  In1 : Inport
  Add1 : Sum
  Add2 : Sum
  Constant : Constant  Value=gps_bias
  Random Source1 : dspsrcs4/Random Source  SrcType=Uniform  MinVal=-gps_ruido  MaxVal=gps_ruido  MeanVal=0  VarVal=1  RepMode=Not repeatable  rawSeed=1  IsInherit=off  SampTime=step_modelo  SampFrame=1  OutComplex=Real  DataType=double  SimulateUsing=Code generation
  Out1 : Outport
  wires:
  Random Source1/1 -> Add2/1
  Constant/1 -> Add1/1
  Add1/1 -> Add2/2
  In1/1 -> Add1/2
  Add2/1 -> Out1/1

== system backups/Sensores Orbital1/Sensor ativado/GPSsensor2 ==
  In1 : Inport
  Add1 : Sum
  Add2 : Sum
  Constant : Constant  Value=gps_bias
  Random Source1 : dspsrcs4/Random Source  SrcType=Uniform  MinVal=-gps_ruido  MaxVal=gps_ruido  MeanVal=0  VarVal=1  RepMode=Not repeatable  rawSeed=1  IsInherit=off  SampTime=step_modelo  SampFrame=1  OutComplex=Real  DataType=double  SimulateUsing=Code generation
  Out1 : Outport
  wires:
  Random Source1/1 -> Add2/1
  Constant/1 -> Add1/1
  Add1/1 -> Add2/2
  In1/1 -> Add1/2
  Add2/1 -> Out1/1

== system backups/atuadoresAtitude/conjunto2TorqRods1RodaReacao/HardwareDeControle (Rodas de Reação + 2 Torqrods) ==
  Tc : Inport
  B_seg : Inport  Port=2
  B_matriz : MATLAB Function  TreatAsAtomicUnit=on
  Demux1 : Demux  Outputs=3
  Gain1 : Gain  Gain=-1
  Gain3 : Gain  Gain=-1
  Inv_B_matriz : MATLAB Function  TreatAsAtomicUnit=on
  MatrixMultiply : Product  Multiplication=Matrix(*)
  MatrixMultiply1 : Product  Multiplication=Matrix(*)
  Mux : Mux  Inputs=3
  Saturation : Saturate  UpperLimit=sat_torquerod  LowerLimit=-sat_torquerod
  Saturation1 : Saturate  UpperLimit=sat_rodareacao  LowerLimit=-sat_rodareacao
  Saturation3 : Saturate  UpperLimit=sat_torquerod  LowerLimit=-sat_torquerod
  rodaReacaoCaracteristicas : Subsystem
  Tc fornecido : Outport  VectorParamsAs1DForOutWhenUnconnected=off
  wires:
  B_matriz/1(y) -> MatrixMultiply1/1
  B_seg/1 -> Inv_B_matriz/1(B_seg), B_matriz/1(B_seg)
  Tc/1 -> MatrixMultiply/2
  MatrixMultiply/1 -> Demux1/1
  Demux1/1 -> Saturation/1  "Mx"
  Demux1/2 -> Saturation1/1  "hwy_dot"
  Demux1/3 -> Saturation3/1  "Mz"
  Saturation/1 -> Mux/1
  Saturation1/1 -> Gain1/1
  Saturation3/1 -> Mux/3
  Mux/1 -> MatrixMultiply1/2
  MatrixMultiply1/1 -> Tc fornecido/1
  Gain1/1 -> rodaReacaoCaracteristicas/1(Tc_entrada)
  rodaReacaoCaracteristicas/1(Tw) -> Gain3/1
  Gain3/1 -> Mux/2
  Inv_B_matriz/1(y) -> MatrixMultiply/1

== system backups/atuadoresAtitude/conjunto2TorqRods1RodaReacao/If Action Subsystem ==
  altSeg : Inport
  latSeg : Inport  Port=2
  lonSeg : Inport  Port=3
  Action Port : ActionPort  ActionPortLabel=if(u1 > 0)
  Gain : Gain  Gain=1e-9
  Gain1 : Gain  Gain=180/pi
  Gain2 : Gain  Gain=180/pi
  World Magnetic Model : aerolibgravity2/World Magnetic Model  model=WMM2020 (2020-2025)  customFile='WMM2020.COF'  units=Metric (MKS)  time_in=off  month=January  day=1  year=2024  action=Error  h_out=off  dec_out=off  inc_out=off  ti_out=off
  Output : Outport
  wires:
  Gain/1 -> Output/1
  altSeg/1 -> World Magnetic Model/1
  lonSeg/1 -> Gain2/1
  Gain1/1 -> World Magnetic Model/2
  latSeg/1 -> Gain1/1
  World Magnetic Model/1 -> Gain/1
  Gain2/1 -> World Magnetic Model/3

== system backups/atuadoresAtitude/conjunto2TorqRods1RodaReacao/If Action Subsystem1 ==
  Action Port : ActionPort  ActionPortLabel=else
  Constant1 : Constant  Value=0  SampleTime=-1
  Constant2 : Constant  Value=0  SampleTime=-1
  Constant5 : Constant  Value=0  SampleTime=-1
  Mux2 : Mux  Inputs=3
  Out1 : Outport
  wires:
  Constant5/1 -> Mux2/3
  Mux2/1 -> Out1/1
  Constant1/1 -> Mux2/1
  Constant2/1 -> Mux2/2

== system backups/atuadoresAtitude/rodaReacao/rodaReacaoCaracteristicas ==
  Tc_entrada : Inport
  Gain : Gain  Gain=1/Km
  Gain2 : Gain  Gain=1/Rm
  Gain3 : Gain  Gain=Km
  Gain4 : Gain  Gain=1/Iw
  Gain5 : Gain  Gain=-1
  Gain6 : Gain  Gain=1/(Ixx+Iyy+Izz)
  Gain7 : Gain  Gain=B
  Gain8 : Gain  Gain=Kv
  Integrator1 : Integrator
  Integrator2 : Integrator
  Limite Corrente : Saturate  UpperLimit=limCorrente  LowerLimit=-limCorrente
  Limite Tensão : Saturate  UpperLimit=limVolt  LowerLimit=-limVolt
  Subsystem : Subsystem
  Sum : Sum  Inputs=|+-
  Sum2 : Sum  Inputs=-+|
  Sum3 : Sum  Inputs=|+-
  Sum4 : Sum  Inputs=-+|
  Tw : Outport
  wires:
  Sum2/1 -> Gain4/1, Gain5/1, Tw/1  "Tw"
  Sum3/1 -> Gain8/1, Gain7/1  "omega_rel"
  Integrator2/1 -> Sum3/2  "omega_b"
  Gain2/1 -> Gain3/1, Sum/2  "im"
  Sum4/1 -> Gain2/1  "V"
  Integrator1/1 -> Sum3/1  "omega_w"
  Gain3/1 -> Sum2/2  "Tm"
  Gain4/1 -> Integrator1/1  "omega_w_dot"
  Gain7/1 -> Sum2/1
  Limite Corrente/1 -> Sum/1
  Tc_entrada/1 -> Gain/1
  Gain/1 -> Limite Corrente/1  "ic"
  Subsystem/1(Voltagem) -> Limite Tensão/1
  Gain8/1 -> Sum4/1
  Gain6/1 -> Integrator2/1  "omega_b_dot"
  Gain5/1 -> Gain6/1  "hb_dot"
  Sum/1 -> Subsystem/1(erroCorrente)  "erroCorrente"
  Limite Tensão/1 -> Sum4/2

== system backups/atuadoresAtitude/rodaReacao/rodaReacaoCaracteristicas1 ==
  Tc_entrada : Inport
  Gain : Gain  Gain=1/Km
  Gain2 : Gain  Gain=1/Rm
  Gain3 : Gain  Gain=Km
  Gain4 : Gain  Gain=1/Iw
  Gain5 : Gain  Gain=-1
  Gain6 : Gain  Gain=1/(Ixx+Iyy+Izz)
  Gain7 : Gain  Gain=B
  Gain8 : Gain  Gain=Kv
  Integrator1 : Integrator
  Integrator2 : Integrator
  Limite Corrente : Saturate  UpperLimit=limCorrente  LowerLimit=-limCorrente
  Limite Tensão : Saturate  UpperLimit=limVolt  LowerLimit=-limVolt
  Subsystem : Subsystem
  Sum : Sum  Inputs=|+-
  Sum2 : Sum  Inputs=-+|
  Sum3 : Sum  Inputs=|+-
  Sum4 : Sum  Inputs=-+|
  Tw : Outport
  wires:
  Limite Tensão/1 -> Sum4/2
  Sum/1 -> Subsystem/1(erroCorrente)  "erroCorrente"
  Gain5/1 -> Gain6/1  "hb_dot"
  Gain6/1 -> Integrator2/1  "omega_b_dot"
  Gain8/1 -> Sum4/1
  Subsystem/1(Voltagem) -> Limite Tensão/1
  Gain/1 -> Limite Corrente/1  "ic"
  Tc_entrada/1 -> Gain/1
  Limite Corrente/1 -> Sum/1
  Gain7/1 -> Sum2/1
  Gain4/1 -> Integrator1/1  "omega_w_dot"
  Gain3/1 -> Sum2/2  "Tm"
  Integrator1/1 -> Sum3/1  "omega_w"
  Sum4/1 -> Gain2/1  "V"
  Gain2/1 -> Sum/2, Gain3/1  "im"
  Integrator2/1 -> Sum3/2  "omega_b"
  Sum3/1 -> Gain7/1, Gain8/1  "omega_rel"
  Sum2/1 -> Tw/1, Gain5/1, Gain4/1  "Tw"

== system backups/atuadoresAtitude/rodaReacao/rodaReacaoCaracteristicas2 ==
  Tc_entrada : Inport
  Gain : Gain  Gain=1/Km
  Gain2 : Gain  Gain=1/Rm
  Gain3 : Gain  Gain=Km
  Gain4 : Gain  Gain=1/Iw
  Gain5 : Gain  Gain=-1
  Gain6 : Gain  Gain=1/(Ixx+Iyy+Izz)
  Gain7 : Gain  Gain=B
  Gain8 : Gain  Gain=Kv
  Integrator1 : Integrator
  Integrator2 : Integrator
  Limite Corrente : Saturate  UpperLimit=limCorrente  LowerLimit=-limCorrente
  Limite Tensão : Saturate  UpperLimit=limVolt  LowerLimit=-limVolt
  Subsystem : Subsystem
  Sum : Sum  Inputs=|+-
  Sum2 : Sum  Inputs=-+|
  Sum3 : Sum  Inputs=|+-
  Sum4 : Sum  Inputs=-+|
  Tw : Outport
  wires:
  Sum2/1 -> Gain4/1, Gain5/1, Tw/1  "Tw"
  Sum3/1 -> Gain8/1, Gain7/1  "omega_rel"
  Integrator2/1 -> Sum3/2  "omega_b"
  Gain2/1 -> Gain3/1, Sum/2  "im"
  Sum4/1 -> Gain2/1  "V"
  Integrator1/1 -> Sum3/1  "omega_w"
  Gain3/1 -> Sum2/2  "Tm"
  Gain4/1 -> Integrator1/1  "omega_w_dot"
  Gain7/1 -> Sum2/1
  Limite Corrente/1 -> Sum/1
  Tc_entrada/1 -> Gain/1
  Gain/1 -> Limite Corrente/1  "ic"
  Subsystem/1(Voltagem) -> Limite Tensão/1
  Gain8/1 -> Sum4/1
  Gain6/1 -> Integrator2/1  "omega_b_dot"
  Gain5/1 -> Gain6/1  "hb_dot"
  Sum/1 -> Subsystem/1(erroCorrente)  "erroCorrente"
  Limite Tensão/1 -> Sum4/2

== system backups/atuadoresAtitude/rodaReacao/rodaReacaoCaracteristicas3 ==
  Tc_entrada : Inport
  Gain : Gain  Gain=1/Km
  Gain2 : Gain  Gain=1/Rm
  Gain3 : Gain  Gain=Km
  Gain4 : Gain  Gain=1/Iw
  Gain5 : Gain  Gain=-1
  Gain6 : Gain  Gain=1/(Ixx+Iyy+Izz)
  Gain7 : Gain  Gain=B
  Gain8 : Gain  Gain=Kv
  Integrator1 : Integrator
  Integrator2 : Integrator
  Limite Corrente : Saturate  UpperLimit=limCorrente  LowerLimit=-limCorrente
  Limite Tensão : Saturate  UpperLimit=limVolt  LowerLimit=-limVolt
  Subsystem : Subsystem
  Sum : Sum  Inputs=|+-
  Sum2 : Sum  Inputs=-+|
  Sum3 : Sum  Inputs=|+-
  Sum4 : Sum  Inputs=-+|
  Tw : Outport
  wires:
  Limite Tensão/1 -> Sum4/2
  Sum/1 -> Subsystem/1(erroCorrente)  "erroCorrente"
  Gain5/1 -> Gain6/1  "hb_dot"
  Gain6/1 -> Integrator2/1  "omega_b_dot"
  Gain8/1 -> Sum4/1
  Subsystem/1(Voltagem) -> Limite Tensão/1
  Gain/1 -> Limite Corrente/1  "ic"
  Tc_entrada/1 -> Gain/1
  Limite Corrente/1 -> Sum/1
  Gain7/1 -> Sum2/1
  Gain4/1 -> Integrator1/1  "omega_w_dot"
  Gain3/1 -> Sum2/2  "Tm"
  Integrator1/1 -> Sum3/1  "omega_w"
  Sum4/1 -> Gain2/1  "V"
  Gain2/1 -> Sum/2, Gain3/1  "im"
  Integrator2/1 -> Sum3/2  "omega_b"
  Sum3/1 -> Gain7/1, Gain8/1  "omega_rel"
  Sum2/1 -> Tw/1, Gain5/1, Gain4/1  "Tw"

== system backups/Atuadores de Atitude/Atuador atitude ativado/Magnetorquer ativado/Conjunto Rodas de Reação + Magnetotorques ==
  note: Entradas
  note: Saídas
  note: Conjunto Rodas de Reação + Magnetotorqueadores
  Tc : Inport
  B_seg : Inport  Port=2
  B_matriz : MATLAB Function  TreatAsAtomicUnit=on
  Demux1 : Demux  Outputs=3
  Gain1 : Gain  Gain=-1
  Gain3 : Gain  Gain=-1
  Inv_B_matriz : MATLAB Function  TreatAsAtomicUnit=on
  MatrixMultiply : Product  Multiplication=Matrix(*)
  MatrixMultiply1 : Product  Multiplication=Matrix(*)
  Model : ModelReference  ModelNameDialog=rodaReacaoCaracteristicas.slx  ModelReferenceVersion=3.129
  Mux : Mux  Inputs=3
  magnetorquerCaracteristicas : ModelReference  ModelNameDialog=magnetorquerCaracteristicas  ModelReferenceVersion=3.127
  magnetorquerCaracteristicas1 : ModelReference  ModelNameDialog=magnetorquerCaracteristicas  ModelReferenceVersion=3.127
  Tc_real : Outport  VectorParamsAs1DForOutWhenUnconnected=off
  wires:
  B_matriz/1(y) -> MatrixMultiply1/1
  MatrixMultiply/1 -> Demux1/1
  Demux1/2 -> Gain1/1  "hwy_dot"
  Demux1/3 -> magnetorquerCaracteristicas1/1  "Mz"
  Mux/1 -> MatrixMultiply1/2
  Gain1/1 -> Model/1
  Model/1 -> Gain3/1
  Gain3/1 -> Mux/2
  Inv_B_matriz/1(y) -> MatrixMultiply/1
  Demux1/1 -> magnetorquerCaracteristicas/1  "Mx"
  magnetorquerCaracteristicas/1 -> Mux/1
  magnetorquerCaracteristicas1/1 -> Mux/3
  Tc/1 -> [Tc]
  [Tc] -> MatrixMultiply/2
  B_seg/1 -> [B_seg]
  [B_seg] -> Inv_B_matriz/1(B_seg), B_matriz/1(B_seg)
  MatrixMultiply1/1 -> [Tc_real]
  [Tc_real] -> Tc_real/1

== system backups/Atuadores de Atitude/Atuador atitude ativado/Magnetorquer ativado/Magnetômetro ==
  B : Inport
  Cast To Single : DataTypeConversion  OutDataTypeStr=single  SaturateOnIntegerOverflow=off  RndMeth=Floor
  Constant : Constant  Value=magne
  If : If  IfExpression=u1 ~= 0
  If Action Subsystem : Subsystem  TreatAsAtomicUnit=on
  If Action Subsystem1 : Subsystem  TreatAsAtomicUnit=on
  Merge : Merge
  B_sen : Outport
  wires:
  Cast To Single/1 -> If/1
  If/2 -> If Action Subsystem1/Action
  If Action Subsystem/1(atitudeSen) -> Merge/1
  If/1 -> If Action Subsystem/Action
  Merge/1 -> B_sen/1
  Constant/1 -> Cast To Single/1
  If Action Subsystem1/1(atitudeSen) -> Merge/2
  B/1 -> If Action Subsystem/1(atitude), If Action Subsystem1/1(atitude)

== system backups/Atuadores de Atitude1/Atuador atitude ativado/Magnetorquer ativado/HardwareDeControle (Rodas de Reação + 2 Torqrods) ==
  Tc : Inport
  B_seg : Inport  Port=2
  B_matriz : MATLAB Function  TreatAsAtomicUnit=on
  Demux1 : Demux  Outputs=3
  Gain1 : Gain  Gain=-1
  Gain3 : Gain  Gain=-1
  Inv_B_matriz : MATLAB Function  TreatAsAtomicUnit=on
  MatrixMultiply : Product  Multiplication=Matrix(*)
  MatrixMultiply1 : Product  Multiplication=Matrix(*)
  Model : ModelReference  ModelNameDialog=rodaReacaoCaracteristicas.slx  ModelReferenceVersion=3.129
  Mux : Mux  Inputs=3
  magnetorquerCaracteristicas : ModelReference  ModelNameDialog=magnetorquerCaracteristicas  ModelReferenceVersion=3.127
  magnetorquerCaracteristicas1 : ModelReference  ModelNameDialog=magnetorquerCaracteristicas  ModelReferenceVersion=3.127
  Tc fornecido : Outport  VectorParamsAs1DForOutWhenUnconnected=off
  wires:
  B_matriz/1(y) -> MatrixMultiply1/1
  B_seg/1 -> Inv_B_matriz/1(B_seg), B_matriz/1(B_seg)
  Tc/1 -> MatrixMultiply/2
  MatrixMultiply/1 -> Demux1/1
  Demux1/2 -> Gain1/1  "hwy_dot"
  Demux1/3 -> magnetorquerCaracteristicas1/1  "Mz"
  Mux/1 -> MatrixMultiply1/2
  MatrixMultiply1/1 -> Tc fornecido/1
  Gain1/1 -> Model/1
  Model/1 -> Gain3/1
  Gain3/1 -> Mux/2
  Inv_B_matriz/1(y) -> MatrixMultiply/1
  Demux1/1 -> magnetorquerCaracteristicas/1  "Mx"
  magnetorquerCaracteristicas/1 -> Mux/1
  magnetorquerCaracteristicas1/1 -> Mux/3

== system backups/Atuadores de Atitude1/Atuador atitude ativado/Magnetorquer ativado/Magnetômetro ==
  B : Inport
  Cast To Single : DataTypeConversion  OutDataTypeStr=single  SaturateOnIntegerOverflow=off  RndMeth=Floor
  Constant : Constant  Value=magne
  If : If  IfExpression=u1 ~= 0
  If Action Subsystem : Subsystem  TreatAsAtomicUnit=on
  If Action Subsystem1 : Subsystem  TreatAsAtomicUnit=on
  Merge : Merge
  B_sen : Outport
  wires:
  Cast To Single/1 -> If/1
  If/2 -> If Action Subsystem1/Action
  If Action Subsystem/1(atitudeSen) -> Merge/1
  If/1 -> If Action Subsystem/Action
  Merge/1 -> B_sen/1
  Constant/1 -> Cast To Single/1
  If Action Subsystem1/1(atitudeSen) -> Merge/2
  B/1 -> If Action Subsystem/1(atitude), If Action Subsystem1/1(atitude)

== system backups/atuadoresAtitude/conjunto2TorqRods1RodaReacao/HardwareDeControle (Rodas de Reação + 2 Torqrods)/rodaReacaoCaracteristicas ==
  Tc_entrada : Inport
  Gain : Gain  Gain=1/Km
  Gain2 : Gain  Gain=1/Rm
  Gain3 : Gain  Gain=Km
  Gain4 : Gain  Gain=1/Iw
  Gain5 : Gain  Gain=-1
  Gain6 : Gain  Gain=1/(Ixx+Iyy+Izz)
  Gain7 : Gain  Gain=B
  Gain8 : Gain  Gain=Kv
  Integrator1 : Integrator
  Integrator2 : Integrator
  Limite Corrente : Saturate  UpperLimit=limCorrente  LowerLimit=-limCorrente
  Limite Tensão : Saturate  UpperLimit=limVolt  LowerLimit=-limVolt
  Subsystem : Subsystem
  Sum : Sum  Inputs=|+-
  Sum2 : Sum  Inputs=-+|
  Sum3 : Sum  Inputs=|+-
  Sum4 : Sum  Inputs=-+|
  Tw : Outport
  wires:
  Sum2/1 -> Gain4/1, Gain5/1, Tw/1  "Tw"
  Sum3/1 -> Gain8/1, Gain7/1  "omega_rel"
  Integrator2/1 -> Sum3/2  "omega_b"
  Gain2/1 -> Gain3/1, Sum/2  "im"
  Sum4/1 -> Gain2/1  "V"
  Integrator1/1 -> Sum3/1  "omega_w"
  Gain3/1 -> Sum2/2  "Tm"
  Gain4/1 -> Integrator1/1  "omega_w_dot"
  Gain7/1 -> Sum2/1
  Limite Corrente/1 -> Sum/1
  Tc_entrada/1 -> Gain/1
  Gain/1 -> Limite Corrente/1  "ic"
  Subsystem/1(Voltagem) -> Limite Tensão/1
  Gain8/1 -> Sum4/1
  Gain6/1 -> Integrator2/1  "omega_b_dot"
  Gain5/1 -> Gain6/1  "hb_dot"
  Sum/1 -> Subsystem/1(erroCorrente)  "erroCorrente"
  Limite Tensão/1 -> Sum4/2

== system backups/atuadoresAtitude/rodaReacao/rodaReacaoCaracteristicas/Subsystem ==
  erroCorrente : Inport
  Controlador Integral : Subsystem
  Voltagem : Outport
  wires:
  Controlador Integral/1(Voltagem) -> Voltagem/1
  erroCorrente/1 -> Controlador Integral/1(Erro na corrente)

== system backups/atuadoresAtitude/rodaReacao/rodaReacaoCaracteristicas1/Subsystem ==
  erroCorrente : Inport
  Controlador Integral : Subsystem
  Voltagem : Outport
  wires:
  erroCorrente/1 -> Controlador Integral/1(Erro na corrente)
  Controlador Integral/1(Voltagem) -> Voltagem/1

== system backups/atuadoresAtitude/rodaReacao/rodaReacaoCaracteristicas2/Subsystem ==
  erroCorrente : Inport
  Controlador Integral : Subsystem
  Voltagem : Outport
  wires:
  Controlador Integral/1(Voltagem) -> Voltagem/1
  erroCorrente/1 -> Controlador Integral/1(Erro na corrente)

== system backups/atuadoresAtitude/rodaReacao/rodaReacaoCaracteristicas3/Subsystem ==
  erroCorrente : Inport
  Controlador Integral : Subsystem
  Voltagem : Outport
  wires:
  erroCorrente/1 -> Controlador Integral/1(Erro na corrente)
  Controlador Integral/1(Voltagem) -> Voltagem/1

== system backups/Atuadores de Atitude/Atuador atitude ativado/Magnetorquer ativado/Magnetômetro/If Action Subsystem ==
  atitude : Inport
  Action Port : ActionPort
  Demux : Demux  Outputs=3
  Mux : Mux  Inputs=3
  magneSensor : Subsystem
  magneSensor1 : Subsystem
  magneSensor2 : Subsystem
  atitudeSen : Outport
  wires:
  Demux/3 -> magneSensor2/1(In1)
  Demux/2 -> magneSensor1/1(In1)
  Demux/1 -> magneSensor/1(In1)
  atitude/1 -> Demux/1
  magneSensor/1(Out1) -> Mux/1  "x"
  magneSensor1/1(Out1) -> Mux/2  "y"
  magneSensor2/1(Out1) -> Mux/3  "z"
  Mux/1 -> atitudeSen/1

== system backups/Atuadores de Atitude/Atuador atitude ativado/Magnetorquer ativado/Magnetômetro/If Action Subsystem1 ==
  atitude : Inport
  Action Port : ActionPort
  atitudeSen : Outport
  wires:
  atitude/1 -> atitudeSen/1

== system backups/Atuadores de Atitude1/Atuador atitude ativado/Magnetorquer ativado/Magnetômetro/If Action Subsystem ==
  atitude : Inport
  Action Port : ActionPort
  Demux : Demux  Outputs=3
  Mux : Mux  Inputs=3
  magneSensor : Subsystem
  magneSensor1 : Subsystem
  magneSensor2 : Subsystem
  atitudeSen : Outport
  wires:
  Demux/3 -> magneSensor2/1(In1)
  Demux/2 -> magneSensor1/1(In1)
  Demux/1 -> magneSensor/1(In1)
  atitude/1 -> Demux/1
  magneSensor/1(Out1) -> Mux/1  "x"
  magneSensor1/1(Out1) -> Mux/2  "y"
  magneSensor2/1(Out1) -> Mux/3  "z"
  Mux/1 -> atitudeSen/1

== system backups/Atuadores de Atitude1/Atuador atitude ativado/Magnetorquer ativado/Magnetômetro/If Action Subsystem1 ==
  atitude : Inport
  Action Port : ActionPort
  atitudeSen : Outport
  wires:
  atitude/1 -> atitudeSen/1

== system backups/atuadoresAtitude/conjunto2TorqRods1RodaReacao/HardwareDeControle (Rodas de Reação + 2 Torqrods)/rodaReacaoCaracteristicas/Subsystem ==
  erroCorrente : Inport
  Controlador Integral : Subsystem
  Voltagem : Outport
  wires:
  Controlador Integral/1(Voltagem) -> Voltagem/1
  erroCorrente/1 -> Controlador Integral/1(Erro na corrente)

== system backups/atuadoresAtitude/rodaReacao/rodaReacaoCaracteristicas/Subsystem/Controlador Integral ==
  Erro na corrente : Inport
  Gain : Gain  Gain=RodKi
  Integrator : Integrator
  Voltagem : Outport  VectorParamsAs1DForOutWhenUnconnected=off
  wires:
  Gain/1 -> Integrator/1
  Erro na corrente/1 -> Gain/1
  Integrator/1 -> Voltagem/1

== system backups/atuadoresAtitude/rodaReacao/rodaReacaoCaracteristicas1/Subsystem/Controlador Integral ==
  Erro na corrente : Inport
  Gain : Gain  Gain=RodKi
  Integrator : Integrator
  Voltagem : Outport  VectorParamsAs1DForOutWhenUnconnected=off
  wires:
  Integrator/1 -> Voltagem/1
  Erro na corrente/1 -> Gain/1
  Gain/1 -> Integrator/1

== system backups/atuadoresAtitude/rodaReacao/rodaReacaoCaracteristicas2/Subsystem/Controlador Integral ==
  Erro na corrente : Inport
  Gain : Gain  Gain=RodKi
  Integrator : Integrator
  Voltagem : Outport  VectorParamsAs1DForOutWhenUnconnected=off
  wires:
  Gain/1 -> Integrator/1
  Erro na corrente/1 -> Gain/1
  Integrator/1 -> Voltagem/1

== system backups/atuadoresAtitude/rodaReacao/rodaReacaoCaracteristicas3/Subsystem/Controlador Integral ==
  Erro na corrente : Inport
  Gain : Gain  Gain=RodKi
  Integrator : Integrator
  Voltagem : Outport  VectorParamsAs1DForOutWhenUnconnected=off
  wires:
  Integrator/1 -> Voltagem/1
  Erro na corrente/1 -> Gain/1
  Gain/1 -> Integrator/1
